simulink model "HW_2_Block_Diagram"  (R2023b)
settings: Solver=VariableStepAuto  StartTime=0.0  StopTime=12  RelTol=1e-3
values from neighbouring files (symbols this model uses):
  b = 5    [HW_2.mat]    (also in HW_2_Test.m = 2; HW_2_a.m = 2; HW_2_a_Rev_1.m = 2)
  gamma = 1    [HW_2.mat]    (also in HW_2_Test.m = 10; HW_2_a.m; HW_2_a_Rev_1.m)
  K = K + dK(k) * dt    [HW_2_Test.m]    (also in HW_2_a.m = K + dKdt(k) * dt; HW_2_a_Rev_1.m = K + dKdt(k) * dt)
settings Model: Creator=hkurt  LastModifiedBy=hkurt

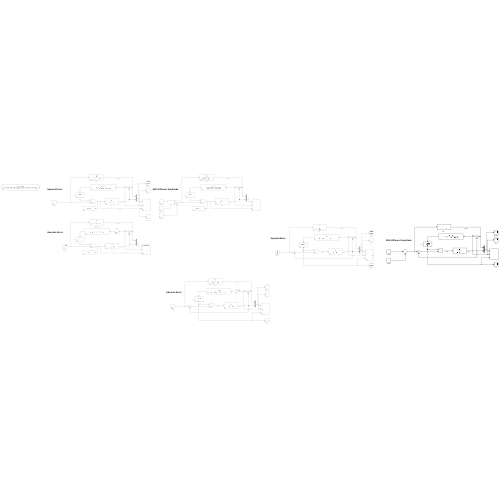
[thumbnail: Simulink's stored preview of the top-level diagram]
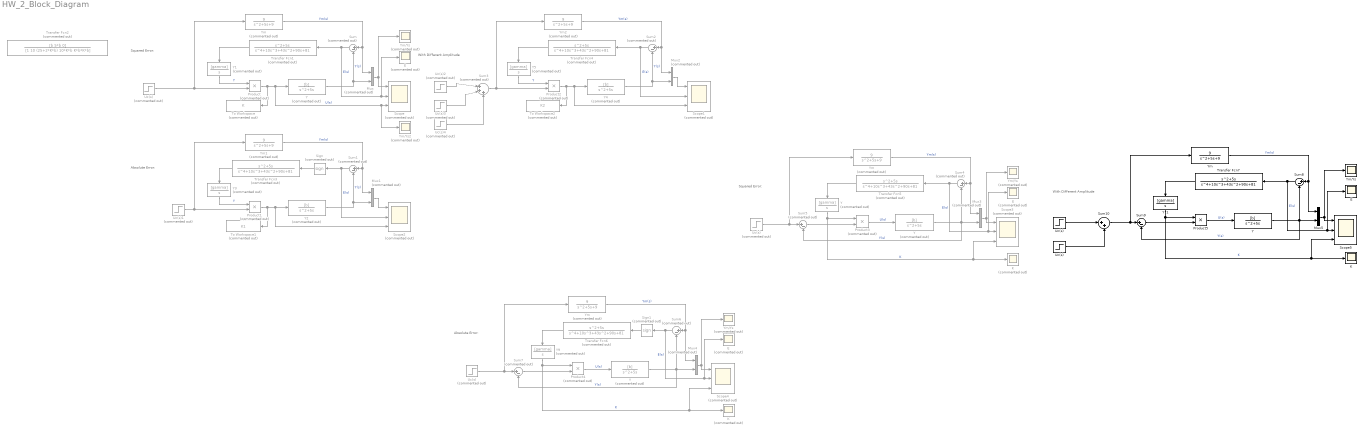
== system HW_2_Block_Diagram ==
  note: Absolute Error:
  note: Squared Error:
  note: With Different Amplitude
  note: Squared Error:
  note: Absolute Error:
  note: With Different Amplitude
  "         Uc(s)        " : Step  Time=5  After=3  SampleTime=0
  " E " : Scope
  " K " : Scope
  " Uc(s)" : Step  SampleTime=0
  " Ym/Ys " : Scope
  E : Scope  Commented=on
  "E " : Scope  Commented=on
  "E  " : Scope  Commented=on
  K : Scope  Commented=on
  "K  " : Scope  Commented=on
  Mux{,1..4} (5 alike) : Mux  Commented=on  Inputs=2
  Mux5 : Mux  Inputs=2
  Product{,1..4} (5 alike) : Product  Commented=on
  Product5 : Product
  Scope{,1..4} (5 alike) : Scope  Commented=on  NumInputPorts=3
  Scope5 : Scope  NumInputPorts=3
  Sign : Signum  Commented=on
  Sign1 : Signum  Commented=on
  Sum{,1..2,4..7} (7 alike) : Sum  Commented=on  Inputs=|+-
  Sum10 : Sum  Inputs=|++
  Sum3 : Sum  Commented=on  Inputs=|+++
  Sum8 : Sum  Inputs=|+-
  Sum9 : Sum  Inputs=|+-
  To Workspace : ToWorkspace  Commented=on  VariableName=K  SaveFormat=Timeseries  SampleTime=-1
  To Workspace1 : ToWorkspace  Commented=on  VariableName=K1  SaveFormat=Timeseries  SampleTime=-1
  To Workspace2 : ToWorkspace  Commented=on  VariableName=K2  SaveFormat=Timeseries  SampleTime=-1
  Transfer Fcn{1,3..6} (5 alike) : TransferFcn  Commented=on  Numerator=[1 5 0]  Denominator=[1 10 43 90 81]
  Transfer Fcn2 : TransferFcn  Commented=on  Numerator=[b 5*b 0]  Denominator=[1 10 (25+2*K*b) 10*K*b K*b*K*b]
  Transfer Fcn7 : TransferFcn  Numerator=[1 5 0]  Denominator=[1 10 43 90 81]
  Uc(s) : Step  Commented=on  SampleTime=0
  "Uc(s) " : Step  Commented=on  SampleTime=0
  "Uc(s)  " : Step  Commented=on  SampleTime=0
  Uc(s)1 : Step  Commented=on  SampleTime=0
  Uc(s)2 : Step  Commented=on  SampleTime=0
  Uc(s)3 : Step  Commented=on  Time=40  After=3  SampleTime=0
  Uc(s)4 : Step  Commented=on  Time=80  After=-1  SampleTime=0
  Y : TransferFcn  Commented=on  Numerator=[b]  Denominator=[1 5 0]
  "Y " : TransferFcn  Commented=on  Numerator=[b]  Denominator=[1 5 0]
  "Y  " : TransferFcn  Commented=on  Numerator=[gamma]  Denominator=[1 0]
  "Y   " : TransferFcn  Commented=on  Numerator=[b]  Denominator=[1 5 0]
  "Y    " : TransferFcn  Numerator=[b]  Denominator=[1 5 0]
  Y  1 : TransferFcn  Numerator=[gamma]  Denominator=[1 0]
  Y{1,3,5,9} (4 alike) : TransferFcn  Commented=on  Numerator=[gamma]  Denominator=[1 0]
  Y2 : TransferFcn  Commented=on  Numerator=[b]  Denominator=[1 5 0]
  Y4 : TransferFcn  Commented=on  Numerator=[b]  Denominator=[1 5 0]
  Ym : TransferFcn  Commented=on  Numerator=[9]  Denominator=[1 5 9]
  "Ym  " : TransferFcn  Commented=on  Numerator=[9]  Denominator=[1 5 9]
  "Ym    " : TransferFcn  Commented=on  Numerator=[9]  Denominator=[1 5 9]
  "Ym     " : TransferFcn  Numerator=[9]  Denominator=[1 5 9]
  Ym/Ys : Scope  Commented=on
  "Ym/Ys " : Scope  Commented=on
  "Ym/Ys  " : Scope  Commented=on
  Ym/Ys2 : Scope  Commented=on
  Ym1 : TransferFcn  Commented=on  Numerator=[9]  Denominator=[1 5 9]
  Ym2 : TransferFcn  Commented=on  Numerator=[9]  Denominator=[1 5 9]
  wires:
  Uc(s)/1 -> Product/2, Ym/1
  Ym/1 -> Mux/1, Sum/1  "Ym(s)"
  Y/1 -> Mux/2, Sum/2  "Y(s)"
  Sum/1 -> Transfer Fcn1/1, E/1, Scope/2  "E(s)"
  Product/1 -> To Workspace/1, Y/1, Ym/Ys2/1, Scope/3  "U(s)"
  Mux/1 -> Scope/1, Ym/Ys/1
  Y1/1 -> Product/1  "Y"
  Transfer Fcn1/1 -> Y1/1
  Uc(s)1/1 -> Product1/2, Ym1/1
  Y3/1 -> Product1/1  "Y"
  Mux1/1 -> Scope2/1
  Y2/1 -> Mux1/2, Sum1/2  "Y(s)"
  Sum1/1 -> Scope2/2, Sign/1  "E(s)"
  Transfer Fcn3/1 -> Y3/1
  Product1/1 -> To Workspace1/1, Scope2/3, Y2/1
  Ym1/1 -> Mux1/1, Sum1/1  "Ym(s)"
  Sign/1 -> Transfer Fcn3/1
  Y5/1 -> Product2/1  "Y"
  Mux2/1 -> Scope1/1
  Y4/1 -> Mux2/2, Sum2/2  "Y(s)"
  Sum2/1 -> Transfer Fcn4/1, Scope1/2  "E(s)"
  Transfer Fcn4/1 -> Y5/1
  Product2/1 -> To Workspace2/1, Y4/1, Scope1/3
  Ym2/1 -> Mux2/1, Sum2/1  "Ym(s)"
  Sum3/1 -> Product2/2, Ym2/1
  Uc(s)2/1 -> Sum3/1
  Uc(s)3/1 -> Sum3/2
  Uc(s)4/1 -> Sum3/3
  Mux3/1 -> "Ym/Ys "/1, Scope3/1
  "Y   "/1 -> Sum4/2, Mux3/2, Sum5/2  "Y(s)"
  Sum4/1 -> Transfer Fcn5/1, "E  "/1, Scope3/2  "E(s)"
  Transfer Fcn5/1 -> "Y  "/1
  "Y  "/1 -> "K  "/1, Scope3/3, Product3/1  "K"
  Product3/1 -> "Y   "/1  "U(s)"
  "Ym    "/1 -> Mux3/1, Sum4/1  "Ym(s)"
  Sum5/1 -> Product3/2
  "Uc(s)  "/1 -> Sum5/1, "Ym    "/1
  Mux4/1 -> "Ym/Ys  "/1, Scope4/1
  "Y "/1 -> Sum6/2, Mux4/2, Sum7/2  "Y(s)"
  Sum6/1 -> Sign1/1, "E "/1, Scope4/2  "E(s)"
  Sum7/1 -> Product4/2
  Product4/1 -> "Y "/1  "U(s)"
  Transfer Fcn6/1 -> Y9/1
  "Uc(s) "/1 -> Sum7/1, "Ym  "/1
  Y9/1 -> K/1, Scope4/3, Product4/1  "K"
  "Ym  "/1 -> Mux4/1, Sum6/1  "Ym(s)"
  Sign1/1 -> Transfer Fcn6/1
  "Y    "/1 -> Sum8/2, Mux5/2, Sum9/2  "Y(s)"
  Sum8/1 -> Transfer Fcn7/1, " E "/1, Scope5/2  "E(s)"
  Sum9/1 -> Product5/2
  Product5/1 -> "Y    "/1  "U(s)"
  Transfer Fcn7/1 -> Y  1/1
  Mux5/1 -> " Ym/Ys "/1, Scope5/1
  Y  1/1 -> " K "/1, Scope5/3, Product5/1  "K"
  "Ym     "/1 -> Mux5/1, Sum8/1  "Ym(s)"
  "         Uc(s)        "/1 -> Sum10/2
  " Uc(s)"/1 -> Sum10/1
  Sum10/1 -> "Ym     "/1, Sum9/1
